simulink model "W04_guidance"  (R2024b)
settings: Solver=ode4  StartTime=0  StopTime=T_final  FixedStep=h  RelTol=1e-3
StopFcn:
  | W04_plot;
values from neighbouring files (symbols this model uses):
  beta_c = 0    [W04_0_setup.m]
  gamma = par(5)    [W04_1_build_guidance.m]
  h = 0.02    [W04_0_setup.m]    (also in W04_1_build_guidance.m = Simulink.Annotation([sub '/note']); W04_1_build_heading.m = add_line(sys, [a; via; b]))
  k_neg = cfg.k_neg    [W04_0_setup.m]    (also in W04_1_build_guidance.m = apar(3);')
  k_pos = cfg.k_pos    [W04_0_setup.m]    (also in W04_1_build_guidance.m = apar(2))
  Kd = 100    [W04_0_setup.m]
  Kp = 300    [W04_0_setup.m]
  mp = 25    [W04_0_setup.m]
  n_min = apar(5)    [W04_1_build_guidance.m]
  R_switch = par(2)    [W04_1_build_guidance.m]
  rp = [0.05 0 -0.35]'    [W04_0_setup.m]
  sw_mode = par(3);'    [W04_1_build_guidance.m]
  V_c = 0    [W04_0_setup.m]
  x0 = zeros(12,1)    [W04_0_setup.m]
  X_ff = 60    [W04_0_setup.m]
  y_pont = cfg.y_pont    [W04_0_setup.m]    (also in W04_1_build_guidance.m = apar(6);')
undefined symbols (not defined in the file or in its folder): animate, Delta, kappa, n_max, WP_E, WP_N
settings Model: Creator=admin  LastModifiedBy=admin
settings DataIOCC: ReturnWorkspaceOutputs=off

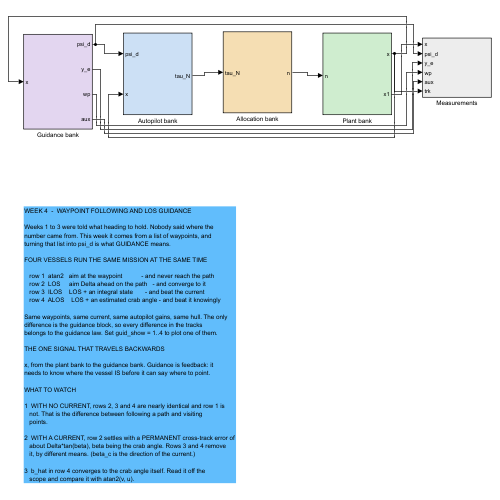
[thumbnail: Simulink's stored preview of the top-level diagram]
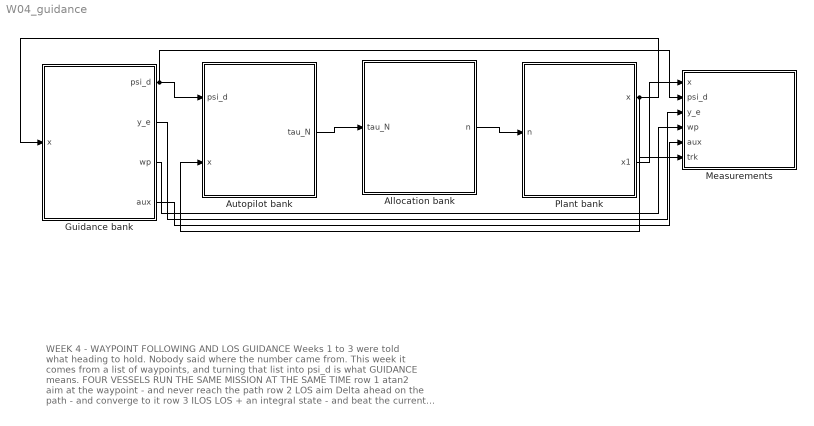
== system W04_guidance ==
  note: WEEK 4  -  WAYPOINT FOLLOWING AND LOS GUIDANCE
      |
      | Weeks 1 to 3 were told what heading to hold. Nobody said where the
      | number came from. This week it comes from a list of waypoints, and
      | turning that list into psi_d is what GUIDANCE means.
      |
      | FOUR VESSELS RUN THE SAME MISSION AT THE SAME TIME
      |
      |    row 1  atan2   aim at the waypoint           - and never reach the path
      |    row 2  LOS     aim Delta ahead on the path   - and converge to it
      |    row 3  ILOS    LOS + an integral state       - and beat the current
      |    row 4  ALOS    LOS + an estimated crab angle - and beat it knowingly
      |
      | Same waypoints, same current, same autopilot gains, same hull. The only
      | difference is the guidance block, so every difference in the tracks
      | belongs to the guidance law. Set guid_show = 1..4 to plot one of them.
      |
      | THE ONE SIGNAL THAT TRAVELS BACKWARDS
      |
      | x, from the plant bank to the guidance bank. Guidance is feedback: it
      | needs to know where the vessel IS before it can say where to point.
      |
      | WHAT TO WATCH
      |
      | 1  WITH NO CURRENT, rows 2, 3 and 4 are nearly identical and row 1 is
      |    not. That is the difference between following a path and visiting
      |    points.
      |
      | 2  WITH A CURRENT, row 2 settles with a PERMANENT cross-track error of
      |    about Delta*tan(beta), beta being the crab angle. Rows 3 and 4 remove
      |    it, by different means. (beta_c is the direction of the current.)
      |
      | 3  b_hat in row 4 converges to the crab angle itself. Read it off the
      |    scope and compare it with atan2(v, u).
  Allocation bank : Subsystem
  Autopilot bank : Subsystem
  Guidance bank : Subsystem
  Measurements : Subsystem
  Plant bank : Subsystem
  wires:
  Guidance bank/1(psi_d) -> Autopilot bank/1(psi_d), Measurements/2(psi_d)
  Plant bank/1(x) -> Guidance bank/1(x), Autopilot bank/2(x), Measurements/6(trk)
  Autopilot bank/1(tau_N) -> Allocation bank/1(tau_N)
  Allocation bank/1(n) -> Plant bank/1(n)
  Plant bank/2(x1) -> Measurements/1(x)
  Guidance bank/2(y_e) -> Measurements/3(y_e)
  Guidance bank/3(wp) -> Measurements/4(wp)
  Guidance bank/4(aux) -> Measurements/5(aux)

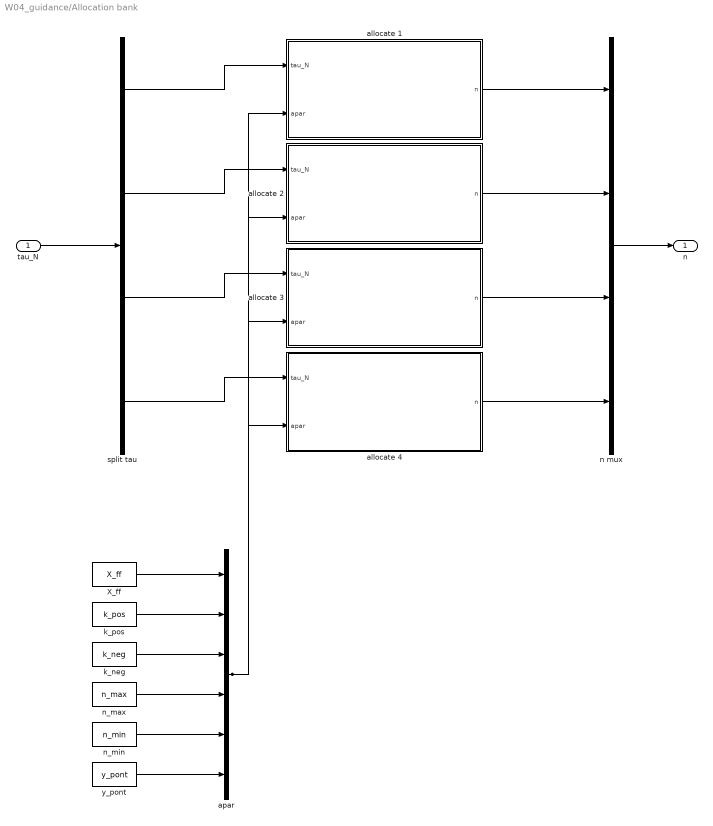
== system W04_guidance/Allocation bank ==
  tau_N : Inport
  X_ff : Constant  Value=X_ff
  allocate 1 : MATLAB Function  TreatAsAtomicUnit=on
  allocate 2 : MATLAB Function  TreatAsAtomicUnit=on
  allocate 3 : MATLAB Function  TreatAsAtomicUnit=on
  allocate 4 : MATLAB Function  TreatAsAtomicUnit=on
  apar : Mux  Inputs=6
  k_neg : Constant  Value=k_neg
  k_pos : Constant  Value=k_pos
  n mux : Mux
  n_max : Constant  Value=n_max
  n_min : Constant  Value=n_min
  split tau : Demux
  y_pont : Constant  Value=y_pont
  n : Outport
  wires:
  X_ff/1 -> apar/1
  k_pos/1 -> apar/2
  k_neg/1 -> apar/3
  n_max/1 -> apar/4
  n_min/1 -> apar/5
  y_pont/1 -> apar/6
  split tau/1 -> allocate 1/1(tau_N)
  apar/1 -> allocate 1/2(apar), allocate 2/2(apar), allocate 3/2(apar), allocate 4/2(apar)
  allocate 1/1(n) -> n mux/1
  split tau/2 -> allocate 2/1(tau_N)
  allocate 2/1(n) -> n mux/2
  split tau/3 -> allocate 3/1(tau_N)
  allocate 3/1(n) -> n mux/3
  split tau/4 -> allocate 4/1(tau_N)
  allocate 4/1(n) -> n mux/4
  tau_N/1 -> split tau/1
  n mux/1 -> n/1

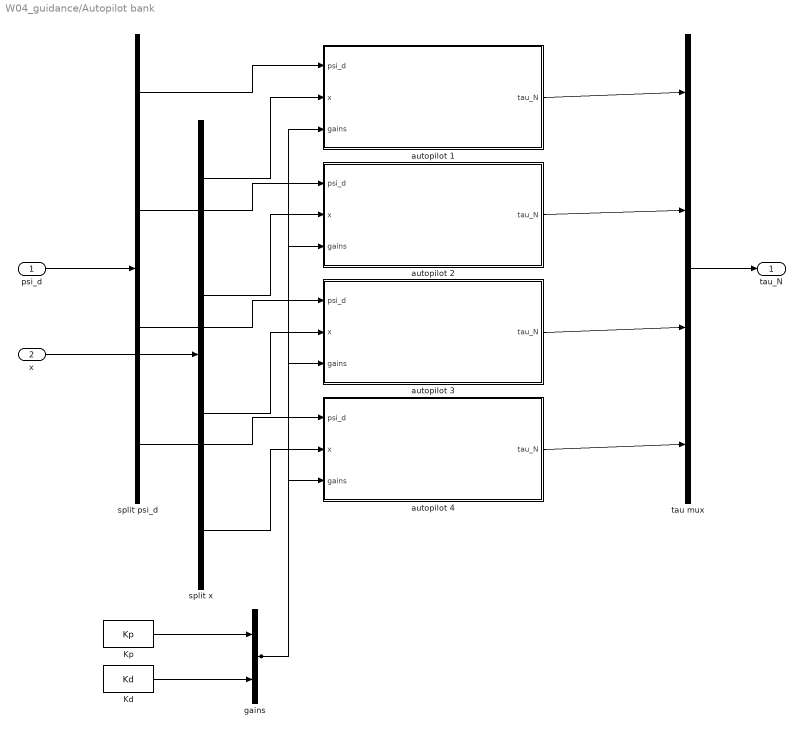
== system W04_guidance/Autopilot bank ==
  psi_d : Inport
  x : Inport  Port=2
  Kd : Constant  Value=Kd
  Kp : Constant  Value=Kp
  autopilot 1 : MATLAB Function  TreatAsAtomicUnit=on
  autopilot 2 : MATLAB Function  TreatAsAtomicUnit=on
  autopilot 3 : MATLAB Function  TreatAsAtomicUnit=on
  autopilot 4 : MATLAB Function  TreatAsAtomicUnit=on
  gains : Mux  Inputs=2
  split psi_d : Demux
  split x : Demux
  tau mux : Mux
  tau_N : Outport
  wires:
  Kp/1 -> gains/1
  Kd/1 -> gains/2
  split psi_d/1 -> autopilot 1/1(psi_d)
  split x/1 -> autopilot 1/2(x)
  gains/1 -> autopilot 1/3(gains), autopilot 2/3(gains), autopilot 3/3(gains), autopilot 4/3(gains)
  autopilot 1/1(tau_N) -> tau mux/1
  split psi_d/2 -> autopilot 2/1(psi_d)
  split x/2 -> autopilot 2/2(x)
  autopilot 2/1(tau_N) -> tau mux/2
  split psi_d/3 -> autopilot 3/1(psi_d)
  split x/3 -> autopilot 3/2(x)
  autopilot 3/1(tau_N) -> tau mux/3
  split psi_d/4 -> autopilot 4/1(psi_d)
  split x/4 -> autopilot 4/2(x)
  autopilot 4/1(tau_N) -> tau mux/4
  psi_d/1 -> split psi_d/1
  x/1 -> split x/1
  tau mux/1 -> tau_N/1

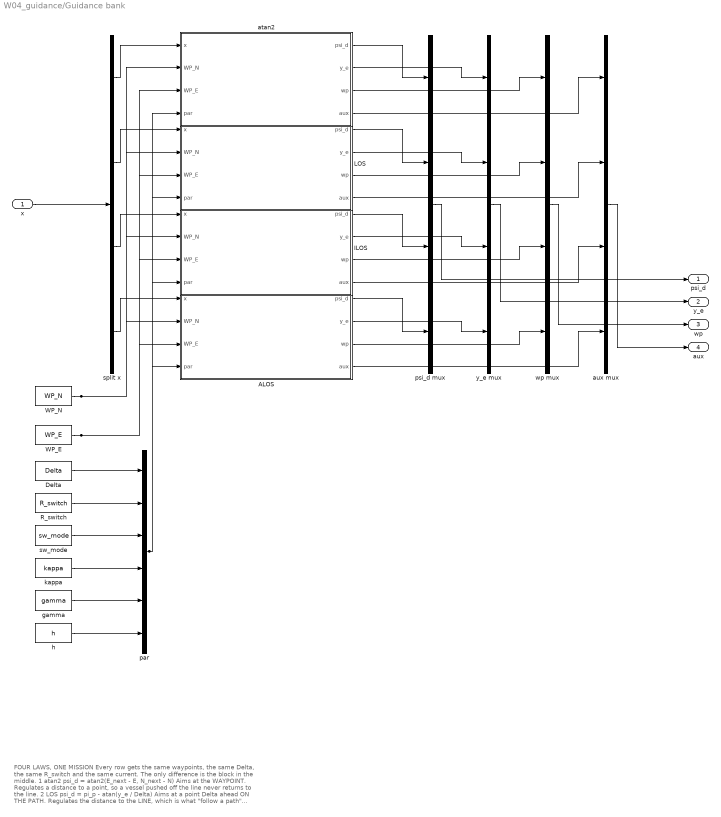
== system W04_guidance/Guidance bank ==
  note: FOUR LAWS, ONE MISSION
      |
      | Every row gets the same waypoints, the same Delta, the same R_switch and
      | the same current. The only difference is the block in the middle.
      |
      |    1  atan2   psi_d = atan2(E_next - E, N_next - N)
      |       Aims at the WAYPOINT. Regulates a distance to a point, so a vessel
      |       pushed off the line never returns to the line.
      |
      |    2  LOS     psi_d = pi_p - atan(y_e / Delta)
      |       Aims at a point Delta ahead ON THE PATH. Regulates the distance to
      |       the LINE, which is what "follow a path" means.
      |
      |    3  ILOS    psi_d = pi_p - atan(y_e/Delta + (kappa/Delta) y_int)
      |       Adds an integral state whose gain SHRINKS as y_e grows, so the
      |       anti-windup is part of the law and not an addition to it.
      |
      |    4  ALOS    psi_d = pi_p - b_hat - atan(y_e / Delta)
      |       Estimates the crab angle itself. b_hat can be read off and compared
      |       with atan2(v, u); an ILOS integral state cannot.
      |
      | Rows 3 and 4 do nothing that row 2 does not, until a current is switched
      | on. That is the experiment of section G.
  x : Inport
  ALOS : MATLAB Function  TreatAsAtomicUnit=on
  Delta : Constant  Value=Delta
  ILOS : MATLAB Function  TreatAsAtomicUnit=on
  LOS : MATLAB Function  TreatAsAtomicUnit=on
  R_switch : Constant  Value=R_switch
  WP_E : Constant  Value=WP_E
  WP_N : Constant  Value=WP_N
  atan2 : MATLAB Function  TreatAsAtomicUnit=on
  aux mux : Mux
  gamma : Constant  Value=gamma
  h : Constant  Value=h
  kappa : Constant  Value=kappa
  par : Mux  Inputs=6
  psi_d mux : Mux
  split x : Demux
  sw_mode : Constant  Value=sw_mode
  wp mux : Mux
  y_e mux : Mux
  psi_d : Outport
  y_e : Outport  Port=2
  wp : Outport  Port=3
  aux : Outport  Port=4
  wires:
  x/1 -> split x/1
  Delta/1 -> par/1
  R_switch/1 -> par/2
  sw_mode/1 -> par/3
  kappa/1 -> par/4
  gamma/1 -> par/5
  h/1 -> par/6
  split x/1 -> atan2/1(x)
  WP_N/1 -> atan2/2(WP_N), LOS/2(WP_N), ILOS/2(WP_N), ALOS/2(WP_N)
  WP_E/1 -> atan2/3(WP_E), LOS/3(WP_E), ILOS/3(WP_E), ALOS/3(WP_E)
  par/1 -> atan2/4(par), LOS/4(par), ILOS/4(par), ALOS/4(par)
  atan2/1(psi_d) -> psi_d mux/1
  atan2/2(y_e) -> y_e mux/1
  atan2/3(wp) -> wp mux/1
  atan2/4(aux) -> aux mux/1
  split x/2 -> LOS/1(x)
  LOS/1(psi_d) -> psi_d mux/2
  LOS/2(y_e) -> y_e mux/2
  LOS/3(wp) -> wp mux/2
  LOS/4(aux) -> aux mux/2
  split x/3 -> ILOS/1(x)
  ILOS/1(psi_d) -> psi_d mux/3
  ILOS/2(y_e) -> y_e mux/3
  ILOS/3(wp) -> wp mux/3
  ILOS/4(aux) -> aux mux/3
  split x/4 -> ALOS/1(x)
  ALOS/1(psi_d) -> psi_d mux/4
  ALOS/2(y_e) -> y_e mux/4
  ALOS/3(wp) -> wp mux/4
  ALOS/4(aux) -> aux mux/4
  psi_d mux/1 -> psi_d/1
  y_e mux/1 -> y_e/1
  wp mux/1 -> wp/1
  aux mux/1 -> aux/1

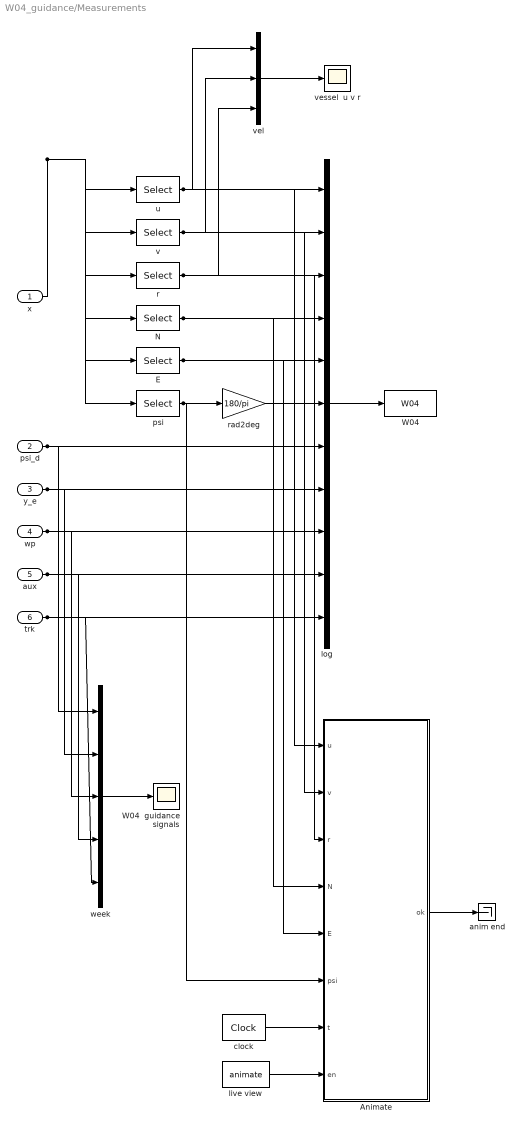
== system W04_guidance/Measurements ==
  x : Inport
  psi_d : Inport  Port=2
  y_e : Inport  Port=3
  wp : Inport  Port=4
  aux : Inport  Port=5
  trk : Inport  Port=6
  Animate : MATLAB Function  TreatAsAtomicUnit=on
  E : Selector  InputPortWidth=12  IndexOptions=Index vector (dialog)  Indices=8  OutputSizes=1
  N : Selector  InputPortWidth=12  IndexOptions=Index vector (dialog)  Indices=7  OutputSizes=1
  W04 : ToWorkspace  VariableName=W04  SaveFormat=Structure With Time  SampleTime=-1
  W04  guidance signals : Scope
  anim end : Terminator
  clock : DigitalClock  SampleTime=h
  live view : Constant  Value=animate
  log : Mux  Inputs=11
  psi : Selector  InputPortWidth=12  IndexOptions=Index vector (dialog)  Indices=12  OutputSizes=1
  r : Selector  InputPortWidth=12  IndexOptions=Index vector (dialog)  Indices=6  OutputSizes=1
  rad2deg : Gain  Gain=180/pi
  u : Selector  InputPortWidth=12  IndexOptions=Index vector (dialog)  Indices=1  OutputSizes=1
  v : Selector  InputPortWidth=12  IndexOptions=Index vector (dialog)  Indices=2  OutputSizes=1
  vel : Mux  Inputs=3
  vessel  u v r : Scope
  week : Mux  Inputs=5
  wires:
  x/1 -> u/1, v/1, r/1, N/1, E/1, psi/1
  log/1 -> W04/1
  psi/1 -> rad2deg/1, Animate/6(psi)
  u/1 -> log/1, vel/1, Animate/1(u)
  v/1 -> log/2, vel/2, Animate/2(v)
  r/1 -> log/3, vel/3, Animate/3(r)
  N/1 -> log/4, Animate/4(N)
  E/1 -> log/5, Animate/5(E)
  rad2deg/1 -> log/6
  psi_d/1 -> log/7, week/1
  y_e/1 -> log/8, week/2
  wp/1 -> log/9, week/3
  aux/1 -> log/10, week/4
  trk/1 -> log/11, week/5
  vel/1 -> vessel  u v r/1
  week/1 -> W04  guidance signals/1
  clock/1 -> Animate/7(t)
  live view/1 -> Animate/8(en)
  Animate/1(ok) -> anim end/1

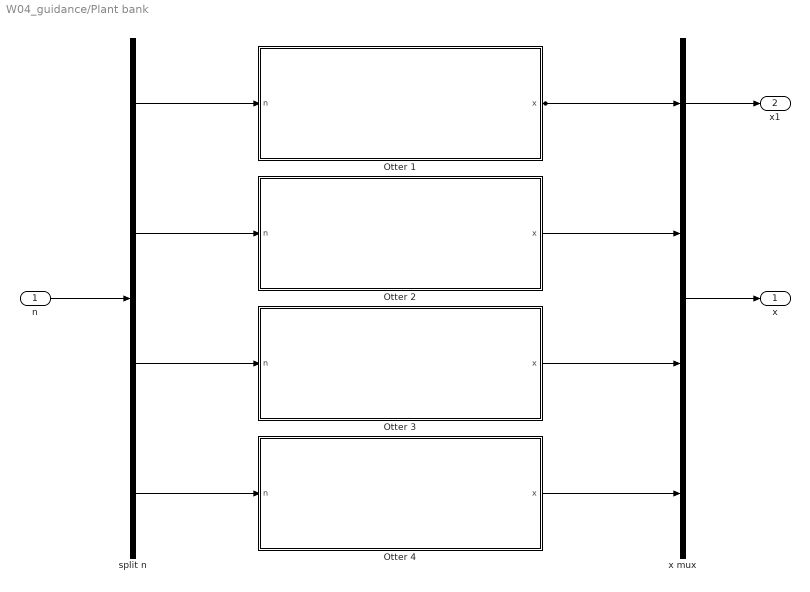
== system W04_guidance/Plant bank ==
  n : Inport
  Otter 1 : Subsystem
  Otter 2 : Subsystem
  Otter 3 : Subsystem
  Otter 4 : Subsystem
  split n : Demux
  x mux : Mux
  x : Outport
  x1 : Outport  Port=2
  wires:
  split n/1 -> Otter 1/1(n)
  Otter 1/1(x) -> x mux/1, x1/1
  split n/2 -> Otter 2/1(n)
  Otter 2/1(x) -> x mux/2
  split n/3 -> Otter 3/1(n)
  Otter 3/1(x) -> x mux/3
  split n/4 -> Otter 4/1(n)
  Otter 4/1(x) -> x mux/4
  n/1 -> split n/1
  x mux/1 -> x/1

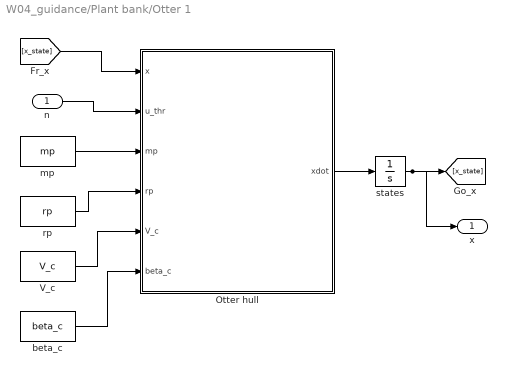
== system W04_guidance/Plant bank/Otter 1 ==
  n : Inport
  Otter hull : MATLAB Function  TreatAsAtomicUnit=on
  V_c : Constant  Value=V_c
  beta_c : Constant  Value=beta_c
  mp : Constant  Value=mp
  rp : Constant  Value=rp
  states : Integrator  InitialCondition=x0
  x : Outport
  wires:
  states/1 -> x/1, [x_state]
  [x_state] -> Otter hull/1(x)
  Otter hull/1(xdot) -> states/1
  beta_c/1 -> Otter hull/6(beta_c)
  V_c/1 -> Otter hull/5(V_c)
  rp/1 -> Otter hull/4(rp)
  mp/1 -> Otter hull/3(mp)
  n/1 -> Otter hull/2(u_thr)

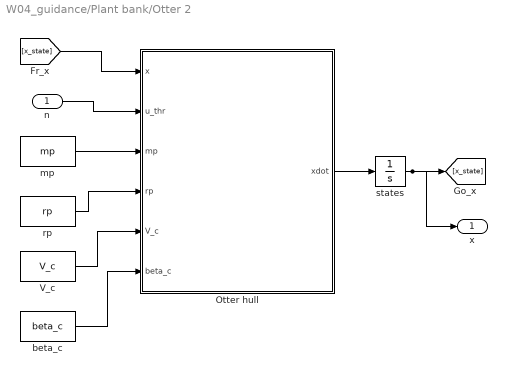
== system W04_guidance/Plant bank/Otter 2 ==
  n : Inport
  Otter hull : MATLAB Function  TreatAsAtomicUnit=on
  V_c : Constant  Value=V_c
  beta_c : Constant  Value=beta_c
  mp : Constant  Value=mp
  rp : Constant  Value=rp
  states : Integrator  InitialCondition=x0
  x : Outport
  wires:
  states/1 -> [x_state], x/1
  [x_state] -> Otter hull/1(x)
  Otter hull/1(xdot) -> states/1
  beta_c/1 -> Otter hull/6(beta_c)
  V_c/1 -> Otter hull/5(V_c)
  rp/1 -> Otter hull/4(rp)
  mp/1 -> Otter hull/3(mp)
  n/1 -> Otter hull/2(u_thr)

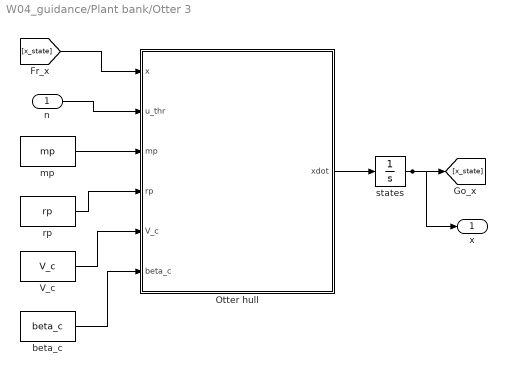
== system W04_guidance/Plant bank/Otter 3 ==
  n : Inport
  Otter hull : MATLAB Function  TreatAsAtomicUnit=on
  V_c : Constant  Value=V_c
  beta_c : Constant  Value=beta_c
  mp : Constant  Value=mp
  rp : Constant  Value=rp
  states : Integrator  InitialCondition=x0
  x : Outport
  wires:
  states/1 -> [x_state], x/1
  [x_state] -> Otter hull/1(x)
  Otter hull/1(xdot) -> states/1
  beta_c/1 -> Otter hull/6(beta_c)
  V_c/1 -> Otter hull/5(V_c)
  rp/1 -> Otter hull/4(rp)
  mp/1 -> Otter hull/3(mp)
  n/1 -> Otter hull/2(u_thr)

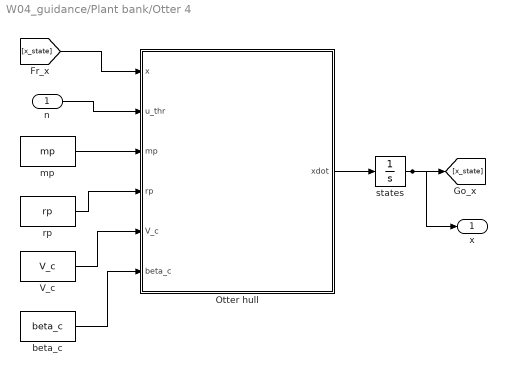
== system W04_guidance/Plant bank/Otter 4 ==
  n : Inport
  Otter hull : MATLAB Function  TreatAsAtomicUnit=on
  V_c : Constant  Value=V_c
  beta_c : Constant  Value=beta_c
  mp : Constant  Value=mp
  rp : Constant  Value=rp
  states : Integrator  InitialCondition=x0
  x : Outport
  wires:
  states/1 -> x/1, [x_state]
  Otter hull/1(xdot) -> states/1
  [x_state] -> Otter hull/1(x)
  beta_c/1 -> Otter hull/6(beta_c)
  V_c/1 -> Otter hull/5(V_c)
  rp/1 -> Otter hull/4(rp)
  mp/1 -> Otter hull/3(mp)
  n/1 -> Otter hull/2(u_thr)

== matlab function W04_guidance/Allocation bank/allocate 1 ==
  data: tau_N input; n output double size=[2 1]; apar input
function n = allocate(tau_N, apar)
%#codegen
% Two demands, two propellers: the map is square and the inverse is unique.
%
%   X = T1 + T2,   N = y_pont (T1 - T2)
%     ==>  T1 = X/2 + N/(2 y_pont),   T2 = X/2 - N/(2 y_pont)
%
% Then the propeller curve is inverted one propeller at a time. Allocating
% THRUST and inverting afterwards is what makes the two shaft speeds come
% out unequal by themselves - see Appendix A1.
X_ff   = apar(1);  k_pos = apar(2);  k_neg  = apar(3);
n_max  = apar(4);  n_min = apar(5);  y_pont = apar(6);

T = [X_ff/2 + tau_N/(2*y_pont);
     X_ff/2 - tau_N/(2*y_pont)];
n = zeros(2,1);
for j = 1:2
    if T(j) >= 0
        nj =  sqrt( T(j) / k_pos);
    else
        nj = -sqrt(-T(j) / k_neg);
    end
    n(j) = min(max(nj, n_min), n_max);
end

== matlab function W04_guidance/Allocation bank/allocate 2 ==
  data: tau_N input; n output double size=[2 1]; apar input
function n = allocate(tau_N, apar)
%#codegen
% Two demands, two propellers: the map is square and the inverse is unique.
%
%   X = T1 + T2,   N = y_pont (T1 - T2)
%     ==>  T1 = X/2 + N/(2 y_pont),   T2 = X/2 - N/(2 y_pont)
%
% Then the propeller curve is inverted one propeller at a time. Allocating
% THRUST and inverting afterwards is what makes the two shaft speeds come
% out unequal by themselves - see Appendix A1.
X_ff   = apar(1);  k_pos = apar(2);  k_neg  = apar(3);
n_max  = apar(4);  n_min = apar(5);  y_pont = apar(6);

T = [X_ff/2 + tau_N/(2*y_pont);
     X_ff/2 - tau_N/(2*y_pont)];
n = zeros(2,1);
for j = 1:2
    if T(j) >= 0
        nj =  sqrt( T(j) / k_pos);
    else
        nj = -sqrt(-T(j) / k_neg);
    end
    n(j) = min(max(nj, n_min), n_max);
end

== matlab function W04_guidance/Allocation bank/allocate 3 ==
  data: tau_N input; n output double size=[2 1]; apar input
function n = allocate(tau_N, apar)
%#codegen
% Two demands, two propellers: the map is square and the inverse is unique.
%
%   X = T1 + T2,   N = y_pont (T1 - T2)
%     ==>  T1 = X/2 + N/(2 y_pont),   T2 = X/2 - N/(2 y_pont)
%
% Then the propeller curve is inverted one propeller at a time. Allocating
% THRUST and inverting afterwards is what makes the two shaft speeds come
% out unequal by themselves - see Appendix A1.
X_ff   = apar(1);  k_pos = apar(2);  k_neg  = apar(3);
n_max  = apar(4);  n_min = apar(5);  y_pont = apar(6);

T = [X_ff/2 + tau_N/(2*y_pont);
     X_ff/2 - tau_N/(2*y_pont)];
n = zeros(2,1);
for j = 1:2
    if T(j) >= 0
        nj =  sqrt( T(j) / k_pos);
    else
        nj = -sqrt(-T(j) / k_neg);
    end
    n(j) = min(max(nj, n_min), n_max);
end

== matlab function W04_guidance/Allocation bank/allocate 4 ==
  data: tau_N input; n output double size=[2 1]; apar input
function n = allocate(tau_N, apar)
%#codegen
% Two demands, two propellers: the map is square and the inverse is unique.
%
%   X = T1 + T2,   N = y_pont (T1 - T2)
%     ==>  T1 = X/2 + N/(2 y_pont),   T2 = X/2 - N/(2 y_pont)
%
% Then the propeller curve is inverted one propeller at a time. Allocating
% THRUST and inverting afterwards is what makes the two shaft speeds come
% out unequal by themselves - see Appendix A1.
X_ff   = apar(1);  k_pos = apar(2);  k_neg  = apar(3);
n_max  = apar(4);  n_min = apar(5);  y_pont = apar(6);

T = [X_ff/2 + tau_N/(2*y_pont);
     X_ff/2 - tau_N/(2*y_pont)];
n = zeros(2,1);
for j = 1:2
    if T(j) >= 0
        nj =  sqrt( T(j) / k_pos);
    else
        nj = -sqrt(-T(j) / k_neg);
    end
    n(j) = min(max(nj, n_min), n_max);
end

== matlab function W04_guidance/Plant bank/Otter 1/Otter hull ==
  data: x input; xdot output double size=[12 1]; u_thr input; mp input; rp input; V_c input; beta_c input
function xdot = otter_hull(x, u_thr, mp, rp, V_c, beta_c)
% Fossen's otter.m, called unchanged from Tools/MSS/VESSELS.
%
%   x       12 states, fed back from the integrator
%   u_thr   propeller shaft speeds [rad/s]
%
% otter.m is not written for code generation, so the call is extrinsic and
% xdot has to be pre-sized for Simulink to know the output width.
coder.extrinsic('otter');

xdot = zeros(12,1);
xdot = otter(x, u_thr, mp, rp, V_c, beta_c);
end

== matlab function W04_guidance/Guidance bank/LOS ==
  settings: updateMethod=DISCRETE  sampleTime=h
  data: x input; psi_d output; WP_N input; WP_E input; par input; y_e output; wp output; aux output
function [psi_d, y_e, wp, aux] = guidance(x, WP_N, WP_E, par)
%#codegen
% One guidance law: waypoint list in, desired heading out.
%
% STATE. k is the active leg, y_int the ILOS integral, b_hat the ALOS
% estimate. They are persistent, which inside a Simulink block means the
% BLOCK owns them: Simulink resets them at the start of every run and two
% blocks never share a copy. That is the difference from calling MSS
% ILOSpsi.m from a script, where one copy is shared by the whole session
% and has to be cleared by hand with "clear ILOSpsi".
persistent k y_int b_hat
if isempty(k), k = 1; y_int = 0; b_hat = 0; end

Delta = par(1);  R_switch = par(2);  sw_mode = par(3);
kappa = par(4);  gamma    = par(5);  h       = par(6);

N = x(7);  E = x(8);
n = numel(WP_N);

% ---- the active leg, and the path-tangential angle -------------------
kn = min(k+1, n);
Nk = WP_N(k);   Ek = WP_E(k);
Nn = WP_N(kn);  En = WP_E(kn);
pi_p = atan2(En - Ek, Nn - Nk);

% ---- along-track and cross-track error, from ONE rotation ------------
%   [x_e]   [ cos pi_p   sin pi_p ] [N - Nk]
%   [y_e] = [-sin pi_p   cos pi_p ] [E - Ek]
dN = N - Nk;  dE = E - Ek;
x_e =  dN*cos(pi_p) + dE*sin(pi_p);
y_e = -dN*sin(pi_p) + dE*cos(pi_p);

% ---- waypoint switching ----------------------------------------------
d = sqrt((Nn-Nk)^2 + (En-Ek)^2);
if sw_mode == 1
    hit = (d - x_e) < R_switch;                   % along-track, as MSS does
else
    hit = sqrt((N-Nn)^2 + (E-En)^2) < R_switch;   % circle of acceptance
end
if hit && k < n-1
    k = k + 1;
end
wp = k;

% ---- LAW 2: LOS - aim at a point Delta ahead ON THE PATH -------------
%   psi_d = pi_p - atan(y_e / Delta)
% Two pieces. pi_p says "line up with the path"; the arctan says "and lean
% towards it by an amount that grows with how far off you are". The
% correction saturates at 90 deg, so the vessel heads almost perpendicular
% to the path when far from it and never turns away from it.
psi_d = pi_p - atan(y_e / Delta);
aux   = 0;

== matlab function W04_guidance/Plant bank/Otter 2/Otter hull ==
  data: x input; xdot output double size=[12 1]; u_thr input; mp input; rp input; V_c input; beta_c input
function xdot = otter_hull(x, u_thr, mp, rp, V_c, beta_c)
% Fossen's otter.m, called unchanged from Tools/MSS/VESSELS.
%
%   x       12 states, fed back from the integrator
%   u_thr   propeller shaft speeds [rad/s]
%
% otter.m is not written for code generation, so the call is extrinsic and
% xdot has to be pre-sized for Simulink to know the output width.
coder.extrinsic('otter');

xdot = zeros(12,1);
xdot = otter(x, u_thr, mp, rp, V_c, beta_c);
end

== matlab function W04_guidance/Plant bank/Otter 3/Otter hull ==
  data: x input; xdot output double size=[12 1]; u_thr input; mp input; rp input; V_c input; beta_c input
function xdot = otter_hull(x, u_thr, mp, rp, V_c, beta_c)
% Fossen's otter.m, called unchanged from Tools/MSS/VESSELS.
%
%   x       12 states, fed back from the integrator
%   u_thr   propeller shaft speeds [rad/s]
%
% otter.m is not written for code generation, so the call is extrinsic and
% xdot has to be pre-sized for Simulink to know the output width.
coder.extrinsic('otter');

xdot = zeros(12,1);
xdot = otter(x, u_thr, mp, rp, V_c, beta_c);
end

== matlab function W04_guidance/Plant bank/Otter 4/Otter hull ==
  data: x input; xdot output double size=[12 1]; u_thr input; mp input; rp input; V_c input; beta_c input
function xdot = otter_hull(x, u_thr, mp, rp, V_c, beta_c)
% Fossen's otter.m, called unchanged from Tools/MSS/VESSELS.
%
%   x       12 states, fed back from the integrator
%   u_thr   propeller shaft speeds [rad/s]
%
% otter.m is not written for code generation, so the call is extrinsic and
% xdot has to be pre-sized for Simulink to know the output width.
coder.extrinsic('otter');

xdot = zeros(12,1);
xdot = otter(x, u_thr, mp, rp, V_c, beta_c);
end

== matlab function W04_guidance/Measurements/Animate ==
  data: u input; ok output; v input; r input; N input; E input; psi input; t input; en input
function ok = Animate(u, v, r, N, E, psi, t, en)
%#codegen
% Live view of the vessel while the model runs.
%
% A MATLAB Function block cannot plot, so the drawing function is declared
% extrinsic: Simulink calls plain MATLAB rather than generating code for it.
% Set animate = 0 in the setup script to switch the live view off.
%
% psi arrives in RADIANS and r in rad/s - the units otter.m works in. The
% wrapper converts them for display, in one place, so no two figures in the
% course can disagree about what a degree is.
coder.extrinsic('W04_animate');
ok = 1;
if en > 0.5
    W04_animate(u, v, r, N, E, psi, t);
end
end

== matlab function W04_guidance/Guidance bank/atan2 ==
  settings: updateMethod=DISCRETE  sampleTime=h
  data: x input; psi_d output; WP_N input; WP_E input; par input; y_e output; wp output; aux output
function [psi_d, y_e, wp, aux] = guidance(x, WP_N, WP_E, par)
%#codegen
% One guidance law: waypoint list in, desired heading out.
%
% STATE. k is the active leg, y_int the ILOS integral, b_hat the ALOS
% estimate. They are persistent, which inside a Simulink block means the
% BLOCK owns them: Simulink resets them at the start of every run and two
% blocks never share a copy. That is the difference from calling MSS
% ILOSpsi.m from a script, where one copy is shared by the whole session
% and has to be cleared by hand with "clear ILOSpsi".
persistent k y_int b_hat
if isempty(k), k = 1; y_int = 0; b_hat = 0; end

Delta = par(1);  R_switch = par(2);  sw_mode = par(3);
kappa = par(4);  gamma    = par(5);  h       = par(6);

N = x(7);  E = x(8);
n = numel(WP_N);

% ---- the active leg, and the path-tangential angle -------------------
kn = min(k+1, n);
Nk = WP_N(k);   Ek = WP_E(k);
Nn = WP_N(kn);  En = WP_E(kn);
pi_p = atan2(En - Ek, Nn - Nk);

% ---- along-track and cross-track error, from ONE rotation ------------
%   [x_e]   [ cos pi_p   sin pi_p ] [N - Nk]
%   [y_e] = [-sin pi_p   cos pi_p ] [E - Ek]
dN = N - Nk;  dE = E - Ek;
x_e =  dN*cos(pi_p) + dE*sin(pi_p);
y_e = -dN*sin(pi_p) + dE*cos(pi_p);

% ---- waypoint switching ----------------------------------------------
d = sqrt((Nn-Nk)^2 + (En-Ek)^2);
if sw_mode == 1
    hit = (d - x_e) < R_switch;                   % along-track, as MSS does
else
    hit = sqrt((N-Nn)^2 + (E-En)^2) < R_switch;   % circle of acceptance
end
if hit && k < n-1
    k = k + 1;
end
wp = k;

% ---- LAW 1: atan2 - aim straight at the next waypoint ----------------
% The obvious answer, and the wrong one. It regulates the DISTANCE TO A
% POINT, not the distance to the LINE, so a vessel pushed off the path
% never comes back to it: it simply approaches the waypoint from wherever
% it happens to be. y_e is still computed, so that the four rows are
% measured with the same yardstick.
psi_d = atan2(En - E, Nn - N);
aux   = 0;

== matlab function W04_guidance/Guidance bank/ILOS ==
  settings: updateMethod=DISCRETE  sampleTime=h
  data: x input; psi_d output; WP_N input; WP_E input; par input; y_e output; wp output; aux output
function [psi_d, y_e, wp, aux] = guidance(x, WP_N, WP_E, par)
%#codegen
% One guidance law: waypoint list in, desired heading out.
%
% STATE. k is the active leg, y_int the ILOS integral, b_hat the ALOS
% estimate. They are persistent, which inside a Simulink block means the
% BLOCK owns them: Simulink resets them at the start of every run and two
% blocks never share a copy. That is the difference from calling MSS
% ILOSpsi.m from a script, where one copy is shared by the whole session
% and has to be cleared by hand with "clear ILOSpsi".
persistent k y_int b_hat
if isempty(k), k = 1; y_int = 0; b_hat = 0; end

Delta = par(1);  R_switch = par(2);  sw_mode = par(3);
kappa = par(4);  gamma    = par(5);  h       = par(6);

N = x(7);  E = x(8);
n = numel(WP_N);

% ---- the active leg, and the path-tangential angle -------------------
kn = min(k+1, n);
Nk = WP_N(k);   Ek = WP_E(k);
Nn = WP_N(kn);  En = WP_E(kn);
pi_p = atan2(En - Ek, Nn - Nk);

% ---- along-track and cross-track error, from ONE rotation ------------
%   [x_e]   [ cos pi_p   sin pi_p ] [N - Nk]
%   [y_e] = [-sin pi_p   cos pi_p ] [E - Ek]
dN = N - Nk;  dE = E - Ek;
x_e =  dN*cos(pi_p) + dE*sin(pi_p);
y_e = -dN*sin(pi_p) + dE*cos(pi_p);

% ---- waypoint switching ----------------------------------------------
d = sqrt((Nn-Nk)^2 + (En-Ek)^2);
if sw_mode == 1
    hit = (d - x_e) < R_switch;                   % along-track, as MSS does
else
    hit = sqrt((N-Nn)^2 + (E-En)^2) < R_switch;   % circle of acceptance
end
if hit && k < n-1
    k = k + 1;
end
wp = k;

% ---- LAW 3: ILOS - an integral state absorbs the current -------------
%   psi_d      = pi_p - atan(Kp y_e + Ki y_int),  Kp = 1/Delta, Ki = kappa Kp
%   d/dt y_int = Delta y_e / (Delta^2 + (y_e + kappa y_int)^2)
% Borhaug, Pavlov and Pettersen (2008). Look at the denominator: the
% integrator gain SHRINKS as y_e grows, so it barely integrates while the
% vessel is still far from the path. That is anti-windup built into the law
% rather than bolted on afterwards - compare Week 2, section F.
Kp = 1 / Delta;
Ki = kappa * Kp;
psi_d = pi_p - atan(Kp*y_e + Ki*y_int);
y_int = y_int + h * Delta*y_e / (Delta^2 + (y_e + kappa*y_int)^2);
aux   = y_int;

== matlab function W04_guidance/Guidance bank/ALOS ==
  settings: updateMethod=DISCRETE  sampleTime=h
  data: x input; psi_d output; WP_N input; WP_E input; par input; y_e output; wp output; aux output
function [psi_d, y_e, wp, aux] = guidance(x, WP_N, WP_E, par)
%#codegen
% One guidance law: waypoint list in, desired heading out.
%
% STATE. k is the active leg, y_int the ILOS integral, b_hat the ALOS
% estimate. They are persistent, which inside a Simulink block means the
% BLOCK owns them: Simulink resets them at the start of every run and two
% blocks never share a copy. That is the difference from calling MSS
% ILOSpsi.m from a script, where one copy is shared by the whole session
% and has to be cleared by hand with "clear ILOSpsi".
persistent k y_int b_hat
if isempty(k), k = 1; y_int = 0; b_hat = 0; end

Delta = par(1);  R_switch = par(2);  sw_mode = par(3);
kappa = par(4);  gamma    = par(5);  h       = par(6);

N = x(7);  E = x(8);
n = numel(WP_N);

% ---- the active leg, and the path-tangential angle -------------------
kn = min(k+1, n);
Nk = WP_N(k);   Ek = WP_E(k);
Nn = WP_N(kn);  En = WP_E(kn);
pi_p = atan2(En - Ek, Nn - Nk);

% ---- along-track and cross-track error, from ONE rotation ------------
%   [x_e]   [ cos pi_p   sin pi_p ] [N - Nk]
%   [y_e] = [-sin pi_p   cos pi_p ] [E - Ek]
dN = N - Nk;  dE = E - Ek;
x_e =  dN*cos(pi_p) + dE*sin(pi_p);
y_e = -dN*sin(pi_p) + dE*cos(pi_p);

% ---- waypoint switching ----------------------------------------------
d = sqrt((Nn-Nk)^2 + (En-Ek)^2);
if sw_mode == 1
    hit = (d - x_e) < R_switch;                   % along-track, as MSS does
else
    hit = sqrt((N-Nn)^2 + (E-En)^2) < R_switch;   % circle of acceptance
end
if hit && k < n-1
    k = k + 1;
end
wp = k;

% ---- LAW 4: ALOS - estimate the crab angle and subtract it -----------
%   psi_d      = pi_p - b_hat - atan(y_e / Delta)
%   d/dt b_hat = gamma Delta y_e / sqrt(Delta^2 + y_e^2)
% Fossen (2023). ILOS absorbs the current into an integral state whose
% value has no physical meaning. ALOS estimates the CRAB ANGLE itself, so
% b_hat converges to a number that can be read off and compared with
% atan2(v, u). Section H checks that it does, and plots the Lyapunov
% function whose derivative the adaptation law was chosen to make negative.
psi_d = pi_p - b_hat - atan(y_e / Delta);
b_hat = b_hat + h * gamma * Delta * y_e / sqrt(Delta^2 + y_e^2);
aux   = b_hat;

== matlab function W04_guidance/Autopilot bank/autopilot 1 ==
  data: psi_d input; tau_N output double size=[1 1]; x input; gains input
function tau_N = autopilot(psi_d, x, gains)
%#codegen
% The Week 3 heading autopilot, unchanged and untuned.
%
%   tau_N = Kp ssa(psi_d - psi) - Kd r
%
% P-D on the heading with the D term acting on the measured yaw RATE, not on
% the derivative of the error. All four rows carry an identical copy, so no
% difference in the results can come from the inner loop.
Kp = gains(1);
Kd = gains(2);

psi = x(12);
r   = x(6);
e   = psi_d - psi;
e   = atan2(sin(e), cos(e));        % ssa: the smallest signed angle
tau_N = Kp * e - Kd * r;

== matlab function W04_guidance/Autopilot bank/autopilot 2 ==
  data: psi_d input; tau_N output double size=[1 1]; x input; gains input
function tau_N = autopilot(psi_d, x, gains)
%#codegen
% The Week 3 heading autopilot, unchanged and untuned.
%
%   tau_N = Kp ssa(psi_d - psi) - Kd r
%
% P-D on the heading with the D term acting on the measured yaw RATE, not on
% the derivative of the error. All four rows carry an identical copy, so no
% difference in the results can come from the inner loop.
Kp = gains(1);
Kd = gains(2);

psi = x(12);
r   = x(6);
e   = psi_d - psi;
e   = atan2(sin(e), cos(e));        % ssa: the smallest signed angle
tau_N = Kp * e - Kd * r;

== matlab function W04_guidance/Autopilot bank/autopilot 3 ==
  data: psi_d input; tau_N output double size=[1 1]; x input; gains input
function tau_N = autopilot(psi_d, x, gains)
%#codegen
% The Week 3 heading autopilot, unchanged and untuned.
%
%   tau_N = Kp ssa(psi_d - psi) - Kd r
%
% P-D on the heading with the D term acting on the measured yaw RATE, not on
% the derivative of the error. All four rows carry an identical copy, so no
% difference in the results can come from the inner loop.
Kp = gains(1);
Kd = gains(2);

psi = x(12);
r   = x(6);
e   = psi_d - psi;
e   = atan2(sin(e), cos(e));        % ssa: the smallest signed angle
tau_N = Kp * e - Kd * r;

== matlab function W04_guidance/Autopilot bank/autopilot 4 ==
  data: psi_d input; tau_N output double size=[1 1]; x input; gains input
function tau_N = autopilot(psi_d, x, gains)
%#codegen
% The Week 3 heading autopilot, unchanged and untuned.
%
%   tau_N = Kp ssa(psi_d - psi) - Kd r
%
% P-D on the heading with the D term acting on the measured yaw RATE, not on
% the derivative of the error. All four rows carry an identical copy, so no
% difference in the results can come from the inner loop.
Kp = gains(1);
Kd = gains(2);

psi = x(12);
r   = x(6);
e   = psi_d - psi;
e   = atan2(sin(e), cos(e));        % ssa: the smallest signed angle
tau_N = Kp * e - Kd * r;
